simulink model "integratoe_derivative"  (R2024b)
settings: Solver=VariableStepAuto  StartTime=0.0  StopTime=10.0  RelTol=1e-3
libraries: simulink x1
settings Model: Creator=vishwanth  LastModifiedBy=vishwanth

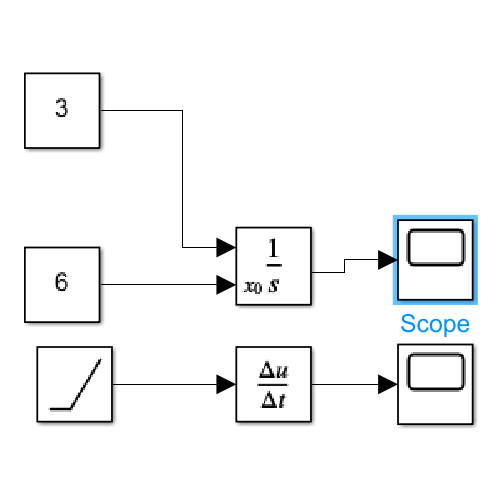
[thumbnail: Simulink's stored preview of the top-level diagram]
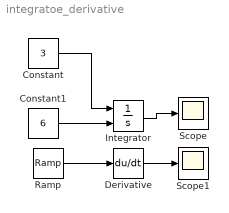
== system integratoe_derivative ==
  Constant : Constant  Value=3
  Constant1 : Constant  Value=6
  Derivative : Derivative
  Integrator : Integrator  InitialConditionSource=external  InitialCondition=2
  Ramp : simulink/Sources/Ramp  slope=0  start=0  InitialOutput=0
  Scope : Scope
  Scope1 : Scope
  wires:
  Constant/1 -> Integrator/1
  Integrator/1 -> Scope/1
  Ramp/1 -> Derivative/1
  Derivative/1 -> Scope1/1
  Constant1/1 -> Integrator/2
